simulink library "AuxEq_Lib"  (R2016b)
settings: Solver=ode45  StartTime=0.0  StopTime=10.0  RelTol=1e-3
values from neighbouring files (symbols this model uses):
  TrimCondition =     [UAV_trimcondition.mat]
libraries: aerolibasang x3, Navigation_Lib x1, simulink x1
settings Model: Creator=Paul Freeman  LastModifiedBy=UAVLAB
settings DataIOCC: LimitDataPoints=on  SaveFormat=Array  SignalLoggingSaveFormat=ModelDataLogs
settings OptimizationCC: BlockReduction=off  BooleanDataType=off  ExpressionDepthLimit=2147483647  LifeSpan=inf
settings DebuggingCC: SaveWithParameterizedLinksMsg=none  UnderspecifiedInitializationDetection=Classic  MergeDetectMultiDrivingBlocksExec=none  SignalResolutionControl=TryResolveAllWithWarning  FcnCallInpInsideContextMsg=warning  StateNameClashWarn=warning  StrictBusMsg=Warning  SFUnexpectedBacktrackingDiag=warning  SFNoUnconditionalDefaultTransitionDiag=warning  SFExecutionAtInitializationDiag=none
settings HardwareCC: ProdBitPerPointer=32  ProdBitPerSizeT=32  ProdBitPerPtrDiffT=32  ProdLargestAtomicFloat=None  ProdIntDivRoundTo=Undefined  ProdEndianess=Unspecified  ProdWordSize=32  ProdHWDeviceType=32-bit Generic  TargetUnknown=on
settings ModelReferenceCC: PropagateSignalLabelsOutOfModel=off
settings GRTTargetCC: TargetLangStandard=C89/C90 (ANSI)  GeneratePreprocessorConditionals=Disable all  CombineOutputUpdateFcns=off  GRTInterface=on
settings ConfigComp: CovMetricSettings=dw  CovHtmlReporting=on  CovSaveCumulativeToWorkspaceVar=on  CovSaveSingleToWorkspaceVar=on  CovExternalEMLEnable=off

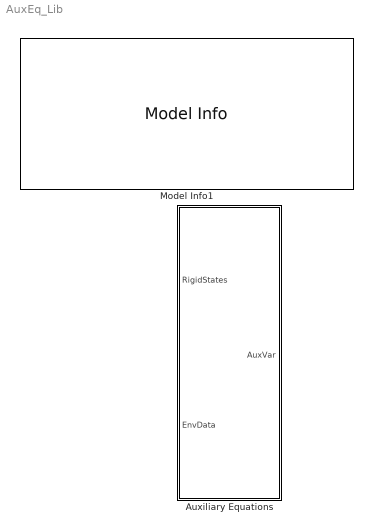
== system AuxEq_Lib ==
  Auxiliary Equations : Subsystem
  Model Info1 : simulink/Model-Wide Utilities/Model Info  BlockCM=None  Frame=on  DisplayStringWithTags=|  HorizontalTextAlignment=Left  LeftAlignmentValue=0.02  SourceBlockDiagram=AuxEq_Lib  TagMaxNumber=20
      | MODEL INFORMATION
      | Auxiliary Equations Library
      | 
      | University of Minnesota
      | Aerospace Engineering and Mechanics
      | Copyright 2011 Regents of the University of Minnesota. All rights reserved.
      | 
      | == SVN Info ==
      | Last modified by %<LastModifiedBy> on %<LastModificationDate>

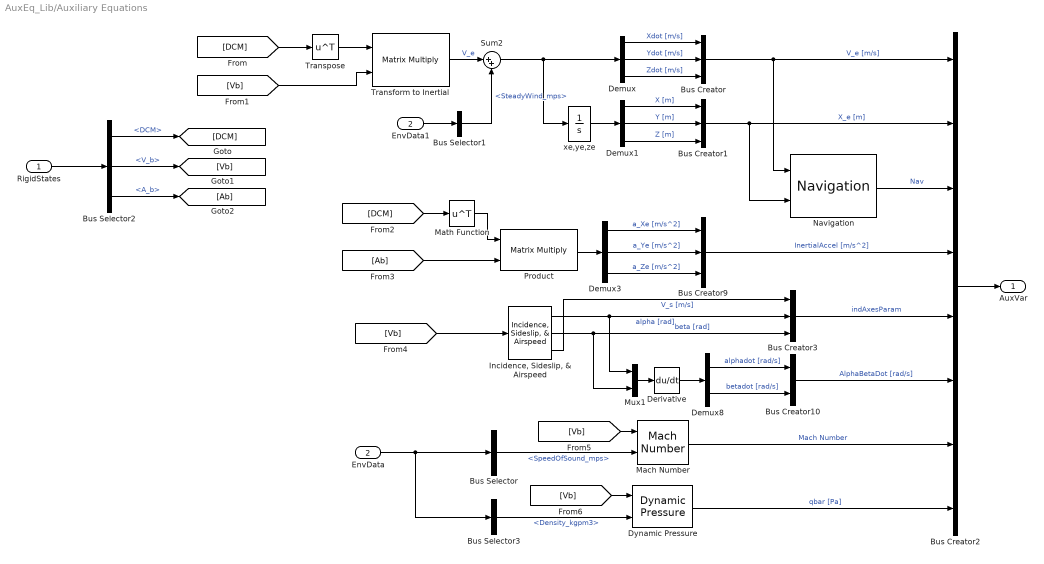
== system AuxEq_Lib/Auxiliary Equations ==
  RigidStates : Inport  OutDataTypeStr=Bus: RigidStates
  EnvData : Inport  Port=2  OutDataTypeStr=Bus: EnvData
  Bus Creator{,1,3,9} (4 alike) : BusCreator  Inputs=3
  Bus Creator10 : BusCreator  Inputs=2
  Bus Creator2 : BusCreator  Inputs=8  OutDataTypeStr=Bus: AuxVar
      settings: InheritFromInputs=off
  Bus Selector : BusSelector  OutputSignals=SpeedOfSound_mps
  Bus Selector1 : BusSelector  OutputSignals=SteadyWind_mps
  Bus Selector2 : BusSelector  OutputSignals=DCM,V_b,A_b
  Bus Selector3 : BusSelector  OutputSignals=Density_kgpm3
  Demux : Demux  Outputs=3
  Demux1 : Demux  Outputs=3
  Demux3 : Demux  Outputs=3
  Demux8 : Demux  Outputs=2
  Derivative : Derivative
  Dynamic Pressure : aerolibasang/Dynamic Pressure
  EnvData1 : InportShadow  Port=2  OutDataTypeStr=Bus: EnvData
  "Incidence, Sideslip, & Airspeed" : aerolibasang/Incidence, Sideslip, & Airspeed
  Mach Number : aerolibasang/Mach Number
  Math Function : Math  Operator=transpose  SaturateOnIntegerOverflow=on
  Mux1 : Mux  Inputs=2
  Navigation : Navigation_Lib/Navigation  Description=|
      | This model produces the followng navigation data for the UAV flight:
      |                                                                     
      | * Geodetic Latitude                                                 
      | * Geodetic Longitude                                                
      | * Geodetic Altitude                                                 
      | * Altitude above Mean Sea Level                                     
      | * Gravitational acceleration vector
  Product : Product  Multiplication=Matrix(*)  RndMeth=Zero
  Sum2 : Sum  Inputs=|++
  Transform to Inertial : Product  Multiplication=Matrix(*)  RndMeth=Zero
  Transpose : Math  Operator=transpose  SaturateOnIntegerOverflow=on
  xe,ye,ze : Integrator  InitialCondition=TrimCondition.InertialIni
  AuxVar : Outport  OutDataTypeStr=Bus: AuxVar
  wires:
  Bus Creator2/1 -> AuxVar/1
  RigidStates/1 -> Bus Selector2/1
  [Vb] -> Mach Number/1
  [Vb] -> "Incidence, Sideslip, & Airspeed"/1
  [DCM] -> Math Function/1
  [Ab] -> Product/2
  Mach Number/1 -> Bus Creator2/7  "Mach Number"
  Demux8/2 -> Bus Creator10/2  "betadot [rad/s]"
  Demux8/1 -> Bus Creator10/1  "alphadot [rad/s]"
  Bus Creator10/1 -> Bus Creator2/6  "AlphaBetaDot [rad/s]"
  Derivative/1 -> Demux8/1
  Mux1/1 -> Derivative/1
  "Incidence, Sideslip, & Airspeed"/3 -> Bus Creator3/1  "V_s [m/s]"
  "Incidence, Sideslip, & Airspeed"/2 -> Bus Creator3/3, Mux1/2  "beta [rad]"
  "Incidence, Sideslip, & Airspeed"/1 -> Bus Creator3/2, Mux1/1  "alpha [rad]"
  Navigation/1 -> Bus Creator2/3  "Nav"
  Bus Creator9/1 -> Bus Creator2/4  "InertialAccel [m/s^2]"
  Demux3/2 -> Bus Creator9/2  "a_Ye [m/s^2]"
  Demux3/3 -> Bus Creator9/3  "a_Ze [m/s^2]"
  Demux3/1 -> Bus Creator9/1  "a_Xe [m/s^2]"
  Product/1 -> Demux3/1
  Math Function/1 -> Product/1
  Bus Selector/1 -> Mach Number/2  "<SpeedOfSound_mps>"
  EnvData/1 -> Bus Selector3/1, Bus Selector/1
  Bus Creator3/1 -> Bus Creator2/5  "indAxesParam"
  Demux1/3 -> Bus Creator1/3  "Z [m]"
  Demux1/2 -> Bus Creator1/2  "Y [m]"
  Demux1/1 -> Bus Creator1/1  "X [m]"
  Bus Creator1/1 -> Bus Creator2/2, Navigation/2  "X_e [m]"
  Demux/3 -> Bus Creator/3  "Zdot [m/s]"
  Demux/2 -> Bus Creator/2  "Ydot [m/s]"
  Demux/1 -> Bus Creator/1  "Xdot [m/s]"
  Bus Creator/1 -> Bus Creator2/1, Navigation/1  "V_e [m/s]"
  Transpose/1 -> Transform to Inertial/1
  [DCM] -> Transpose/1
  EnvData1/1 -> Bus Selector1/1
  Transform to Inertial/1 -> Sum2/1  "V_e"
  Bus Selector1/1 -> Sum2/2  "<SteadyWind_mps>"
  Sum2/1 -> Demux/1, xe,ye,ze/1
  xe,ye,ze/1 -> Demux1/1
  Bus Selector2/1 -> [DCM]  "<DCM>"
  Bus Selector2/2 -> [Vb]  "<V_b>"
  Bus Selector2/3 -> [Ab]  "<A_b>"
  [Vb] -> Transform to Inertial/2
  [Vb] -> Dynamic Pressure/1
  Bus Selector3/1 -> Dynamic Pressure/2  "<Density_kgpm3>"
  Dynamic Pressure/1 -> Bus Creator2/8  "qbar [Pa]"
